simulink model "SubSystemLed"  (R2016b)
settings: Solver=FixedStepDiscrete  StartTime=0.0  StopTime=10000  FixedStep=.0001  RelTol=1e-3
libraries: simulink x1
settings Model: Creator=3essawy  LastModifiedBy=3essawy
settings OptimizationCC: DefaultParameterBehavior=Inlined
settings DebuggingCC: ParameterTunabilityLossMsg=error
settings RTWCC: SystemTargetFile=ert.tlc  GenCodeOnly=on  TemplateMakefile=ert_default_tmf  Description=Embedded Coder  GenerateReport=on  IncludeHyperlinkInReport=on  LaunchReport=on  GenerateTraceInfo=on  GenerateTraceReport=on  GenerateTraceReportSl=on  GenerateTraceReportSf=on  GenerateTraceReportEml=on
settings CodeAppCC: ForceParamTrailComments=on  IgnoreCustomStorageClasses=off  OperatorAnnotations=on  SimulinkDataObjDesc=on  SFDataObjDesc=on  MATLABFcnDesc=on  InsertBlockDesc=on  MATLABSourceComments=on
settings ERTTargetCC: TargetLangStandard=C99 (ISO)  GenerateSampleERTMain=on  InlinedParameterPlacement=NonHierarchical  ERTCustomFileTemplate=example_file_process.tlc  EnableUserReplacementTypes=on

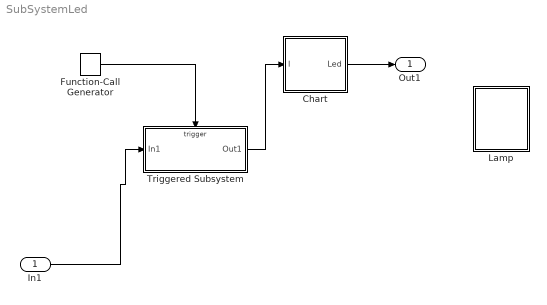
== system SubSystemLed ==
  In1 : Inport
  Chart : Stateflow chart  TreatAsAtomicUnit=on
  Function-Call Generator : simulink/Ports & Subsystems/Function-Call Generator  sample_time=5  numberOfIterations=1
  Lamp : Subsystem  DialogController=hmiCreateDDGDialog  IsWebBlock=on  mask(MWDashboardBlock){webBlockId=670d4ece-7629-422c-b3a4-8ab22eb7463f, webBlockType=lamp, ShowInLibBrowser=on, ShowInitialText=on, HMISrcModelName=SubSystemLed}
      mask prompts: webBlockType "WebBlock Type"; HMISrcModelName "Source Model"
      mask help: SimulinkHMI:dialogs:LampDialogDesc
      mask Help: helpview([docroot '/mapfiles/simulink.map'], 'hmi_lamp')
      mask Display:
      | if strcmp(get_param(bdroot(gcb),'BlockDiagramType'), 'library')
      |     image([(matlabroot) '/toolbox/simulink/hmi/icons/Lamp.png']);
      | end
  Triggered Subsystem : Subsystem  TreatAsAtomicUnit=on
  Out1 : Outport
  wires:
  Triggered Subsystem/1(Out1) -> Chart/1(I)
  Function-Call Generator/1 -> Triggered Subsystem/Trigger
  In1/1 -> Triggered Subsystem/1(In1)
  Chart/1(Led) -> Out1/1

== system SubSystemLed/Lamp ==

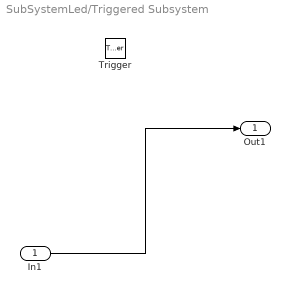
== system SubSystemLed/Triggered Subsystem ==
  In1 : Inport
  Trigger : TriggerPort  TriggerType=function-call  VariantControl=Variant  StatesWhenEnabling=reset
  Out1 : Outport
  wires:
  In1/1 -> Out1/1

== stateflow chart SubSystemLed/Chart ==
  (default) -> (junction 7)
  (junction 7) -> (junction 8) [order 1] : [I>0]
  (junction 7) -> (junction 9) [order 2] : {Led=0;}
  (junction 8) -> (junction 10) : {Led=1;}
  (junction 10) -> (junction 9)
  (junction 9) -> (junction 11)
  data: Led output; I input
